simulink model "q2_b2"  (R2022a)
settings: Solver=VariableStepAuto  StartTime=0.0  StopTime=25  RelTol=1e-3
settings Model: Creator=Aref  LastModifiedBy=ZahraIranpour
settings SolverCC: AlgebraicLoopSolver=TrustRegion
settings DataIOCC: ReturnWorkspaceOutputs=off
settings DebuggingCC: UnconnectedInputMsg=warning  UnconnectedOutputMsg=warning  UnconnectedLineMsg=warning  SFMachineParentedDataDiag=warning  ArithmeticOperatorsInVariantConditions=warning
settings SFSimCC: CustomCodeUndefinedFunction=UseInterfaceOnly

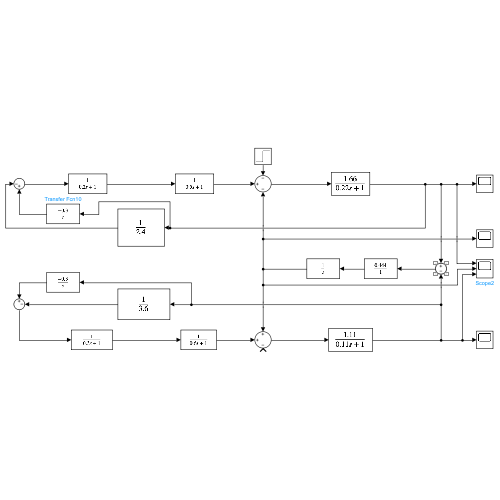
[thumbnail: Simulink's stored preview of the top-level diagram]
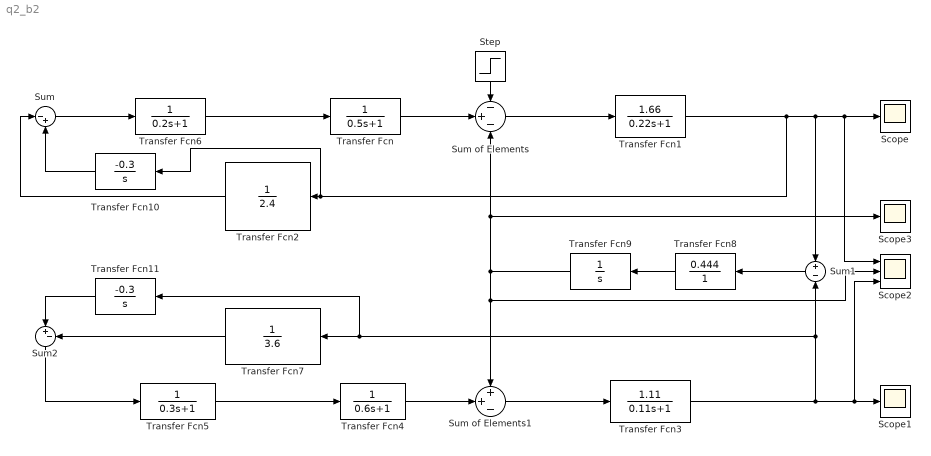
== system q2_b2 ==
  Scope : Scope
  Scope1 : Scope
  Scope2 : Scope  NumInputPorts=3
  Scope3 : Scope
  Step : Step  After=0.15  SampleTime=0
  Sum : Sum  Inputs=|-+
  Sum of Elements : Sum  Inputs=-+-
  Sum of Elements1 : Sum  Inputs=++-
  Sum1 : Sum  Inputs=+-
  Sum2 : Sum  Inputs=|+-
  Transfer Fcn : TransferFcn  Denominator=[0.5 1]
  Transfer Fcn1 : TransferFcn  Numerator=[1.66]  Denominator=[0.22 1]
  Transfer Fcn10 : TransferFcn  Numerator=[-0.3]  Denominator=[1 0]
  Transfer Fcn11 : TransferFcn  Numerator=[-0.3]  Denominator=[1 0]
  Transfer Fcn2 : TransferFcn  Denominator=[2.4]
  Transfer Fcn3 : TransferFcn  Numerator=[1.11]  Denominator=[0.11 1]
  Transfer Fcn4 : TransferFcn  Denominator=[0.6 1]
  Transfer Fcn5 : TransferFcn  Denominator=[0.3 1]
  Transfer Fcn6 : TransferFcn  Denominator=[0.2 1]
  Transfer Fcn7 : TransferFcn  Denominator=[3.6]
  Transfer Fcn8 : TransferFcn  Numerator=[0.444]  Denominator=[0 1]
  Transfer Fcn9 : TransferFcn  Denominator=[1 0]
  wires:
  Sum of Elements/1 -> Transfer Fcn1/1
  Transfer Fcn/1 -> Sum of Elements/2
  Step/1 -> Sum of Elements/1
  Transfer Fcn5/1 -> Transfer Fcn4/1
  Transfer Fcn4/1 -> Sum of Elements1/2
  Transfer Fcn6/1 -> Transfer Fcn/1
  Sum of Elements1/1 -> Transfer Fcn3/1
  Transfer Fcn7/1 -> Sum2/2
  Sum2/1 -> Transfer Fcn5/1
  Sum1/1 -> Transfer Fcn8/1
  Transfer Fcn8/1 -> Transfer Fcn9/1
  Transfer Fcn9/1 -> Scope2/2, Sum of Elements1/1, Scope3/1, Sum of Elements/3
  Transfer Fcn2/1 -> Sum/1
  Sum/1 -> Transfer Fcn6/1
  Transfer Fcn10/1 -> Sum/2
  Transfer Fcn1/1 -> Scope/1, Scope2/1, Sum1/1, Transfer Fcn10/1, Transfer Fcn2/1
  Transfer Fcn11/1 -> Sum2/1
  Transfer Fcn3/1 -> Scope1/1, Scope2/3, Sum1/2, Transfer Fcn11/1, Transfer Fcn7/1
